simulink model "scudder"  (Simulink 2.09)
settings: Solver=ode45  StartTime=0.0  StopTime=0.4  RelTol=1e-5  AbsTol=1e-8
libraries: simulink x1
settings Model: ConsistencyChecking=off

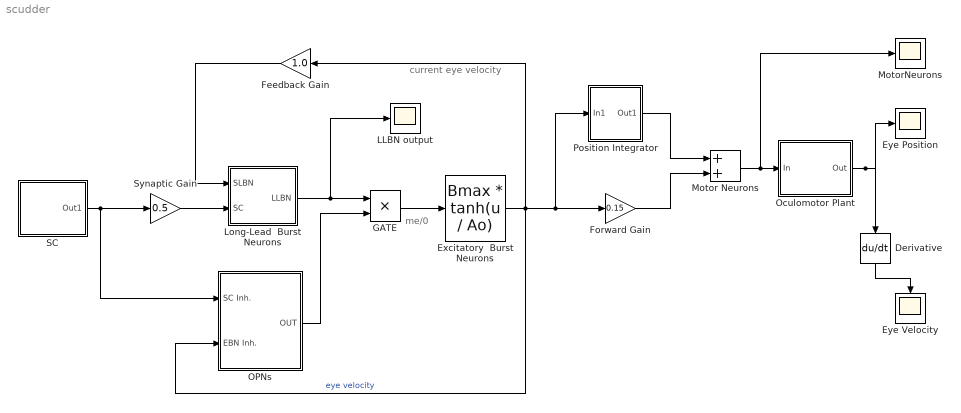
== system scudder ==
  note: current eye velocity
  note: me/0
  Derivative : Derivative  Orientation=down
  Excitatory  Burst Neurons : Fcn  Expr=Bmax * tanh(u / Ao)  mask(Burstcell Nonlinearity){Bmax=700, Ao=7}
      mask prompts: Bmax "Asymptote (Bmax): deg/s"; Ao "Angular Constant (Ao): deg"
      mask help:
      | Function:
      |        B = Bmax * tanh (me / Ao)
      |
      |     Parameters:  Bmax (deg/s)
      |                           Ao (deg)
      mask Help:
      | Bmax is the maximal firing frequency of the burst cells (expressed in deg/sec)
      |           It corresponds to the asymptote of the main sequence.
      | 
      | Ao     is the `angular constant' (in deg), which is a measure of the steepness of              the main  sequence curve for saccades.
      mask Display:
      | plot([0 1],[.5 .5]) plot([.5 .5],[0 1])
      | plot([0 .1 .2 .3 .4 .5 .6 .7 .8 .9 1],[ 0 0 .07 .17 .32 .5 .68 .83 .93 1 1])
      | text(.4,.8,'B') text(.8,.3,'me')
  Eye Position : Scope
      settings: TickLabels=on  TimeRange=auto  YMin=-10  YMax=50  SaveToWorkspace=off  SaveName=ScopeData
  Eye Velocity : Scope
      settings: Orientation=down  TickLabels=on  TimeRange=auto  YMin=-50  YMax=700  SaveToWorkspace=off  SaveName=ScopeData
  "Feedback Gain " : Gain  Orientation=left  Gain=1.0
  Forward Gain : Gain  Gain=0.15
  GATE : Product  Inputs=2
  LLBN output : Scope
      settings: TickLabels=on  TimeRange=auto  YMin=-5  YMax=20  SaveToWorkspace=off  SaveName=ScopeData
  Long-Lead  Burst Neurons : Subsystem
      mask Type: Long-Lead Burst Neurons
      mask Description: Comparator that integrates the difference between a desired eye velocity signal  from the Superior Colliculus, and the current eye velocity from the Short-Lead Burst Neurons.
      mask Display:
      | text(0.5,0.5,'LLBN')
      | text(0.05,0.8,'- slbn')
      | text(0.05,0.2,'+ SC')
  Motor Neurons : Sum  Inputs=++
  MotorNeurons : Scope
      settings: TickLabels=on  TimeRange=auto  YMin=-10  YMax=150  SaveToWorkspace=off  SaveName=ScopeData
  "OPNs " : Subsystem  mask(OPNs){DEL=15, G=0.2, bias=80}
      mask prompts: DEL "Trigger Delay (ms)"; G "SC Gain"; bias "BIAS  (Hz)"
      mask help:
      | Pause system that triggers eye by an attenuated SC input burst, and inhibits the burst generator during fixations with intensity Bias.
      | During the saccade, the burst generator inhibits the pause cells.
      mask Help:
      | User controls:
      |         Bias level (in Hz)   (defines the Pause neuron activity level during fixation)
      |         SC burst, of which the Gain can be set.
      |          Trigger delay (in ms), which determines saccade onset (and kinematics!)
      | Inputs:
      |         SC burst, attenuated by OPN inhibition gain, and delayed.
      |         Horizontal eye velocity (5ms latch delay)
      | Outputs:
      |          either 0 or 1
      mask Display:
      | plot([.1 .3],[.4 .4])
      | plot([.3 .5],[.4 .6])
      | plot([.5 .65],[.4 .4])
      | text(.65,.65,'0')
      | text(.57,.40,'me')
      | 
      | plot([.1 .7],[.3 .3])  plot([.1 .1],[.3 .7])
      | plot([.1 .7],[.7 .7])  plot([.7 .7],[.3 .7])
  Oculomotor Plant : Subsystem  mask(Oculomotor Plant){T1=0.15, T2=0.020}
      mask prompts: T1 "High Time Constant (T1)"; T2 "Low Time Constant (T2)"
      mask help:
      | Second order model of the oculomotor plant
      | as proposed by Robinson and colleagues.
      |
      |  Model equation in Laplace notation:
      |
      |                         1
      |  H(s) = ---------------
      |             (1 + s.T1) . (1 + s.T2)
      mask Help:
      | T1 is the `high' time constant (muscle twitch relaxation time)
      |       default value: 0.15 sec
      |  T2 is the `low' time constant (muscle twitch contraction time)
      |       default value: 0.012 sec
      mask Display:
      | plot([0 0.1 0.15 0.2 0.25 0.3 0.5 0.7 0.9 1], [0 0.1 0.4 0.65 0.66 0.55 0.35 0.15 0.05 0])
      | text(0.04,0.5,'T2') text(0.55,0.5, 'T1')
  Position Integrator : Subsystem  mask(Eye Position Integrator){G=1.0}
      mask prompts: G "Integrator Gain"
      mask Display: text(.35,.5,'INT')
  "SC " : Subsystem  mask{FR=800, D=50}
      mask prompts: FR "Firing Rate (FR, in Hz)"; D "Burst Duration (D,  in msec)"
      mask help: The Superior Colliculus issues a burst of spikes of height FR (Hz) and duration D (in sec).
      mask Display:
      | text(.2,.85,'SC BURST')
      | plot([.2 .35,.36,.65,.66,.8],[.05,.05,.5,.5,.05,.05])
      | text(.15,.5,'FR')
      | text(.5,.05,'D')
  Synaptic Gain : Gain  Gain=0.5
  wires:
  "SC "/1(Out1) -> "OPNs "/1(SC Inh.), Synaptic Gain/1
  Derivative/1 -> Eye Velocity/1
  Oculomotor Plant/1(Out) -> Derivative/1, Eye Position/1
  Long-Lead  Burst Neurons/1(LLBN) -> LLBN output/1, GATE/1
  GATE/1 -> Excitatory  Burst Neurons/1
  "Feedback Gain "/1 -> Long-Lead  Burst Neurons/1(SLBN)
  "OPNs "/1(OUT) -> GATE/2
  Excitatory  Burst Neurons/1 -> "Feedback Gain "/1, "OPNs "/2(EBN Inh.), Position Integrator/1(In1), Forward Gain/1  "eye velocity"
  Synaptic Gain/1 -> Long-Lead  Burst Neurons/2(SC)
  Position Integrator/1(Out1) -> Motor Neurons/1
  Forward Gain/1 -> Motor Neurons/2
  Motor Neurons/1 -> MotorNeurons/1, Oculomotor Plant/1("In ")

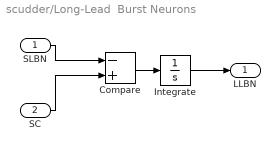
== system scudder/Long-Lead  Burst Neurons ==
  SLBN : Inport  Port=1  PortWidth=-1  SampleTime=-1
  SC : Inport  Port=2  PortWidth=-1  SampleTime=-1
  "Compare " : Sum  Inputs=-+
  Integrate : Integrator  ExternalReset=none  InitialConditionSource=internal  InitialCondition=0  LimitOutput=off  UpperSaturationLimit=inf  LowerSaturationLimit=-inf  ShowSaturationPort=off  ShowStatePort=off  AbsoluteTolerance=auto
  LLBN : Outport  Port=1  InitialOutput=0
  wires:
  SC/1 -> "Compare "/2
  Integrate/1 -> LLBN/1
  SLBN/1 -> "Compare "/1
  "Compare "/1 -> Integrate/1

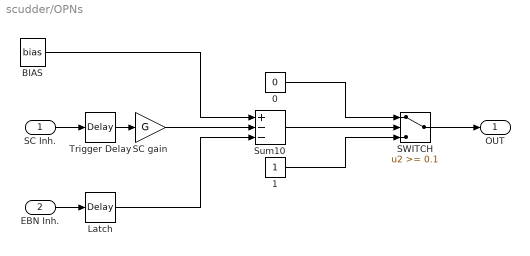
== system scudder/OPNs  ==
  SC Inh. : Inport  Port=1  PortWidth=-1  SampleTime=-1
  EBN Inh. : Inport  Port=2  PortWidth=-1  SampleTime=-1
  0 : Constant  Value=0
  1 : Constant  Value=1
  BIAS : Constant  Value=bias
  Latch : TransportDelay  DelayTime=0.005  InitialInput=0  BufferSize=1024
  SC gain : Gain  Gain=G
  SWITCH : Switch  Threshold=0.1
  Sum10 : Sum  Inputs=+--
  Trigger Delay : TransportDelay  DelayTime=0.001*DEL  InitialInput=0  BufferSize=1024
  OUT : Outport  Port=1  InitialOutput=0
  wires:
  EBN Inh./1 -> Latch/1
  Latch/1 -> Sum10/3
  Trigger Delay/1 -> SC gain/1
  SC Inh./1 -> Trigger Delay/1
  SC gain/1 -> Sum10/2
  Sum10/1 -> SWITCH/2
  1/1 -> SWITCH/3
  0/1 -> SWITCH/1
  SWITCH/1 -> OUT/1
  BIAS/1 -> Sum10/1

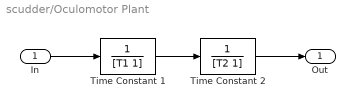
== system scudder/Oculomotor Plant ==
  "In " : Inport  Port=1  PortWidth=-1  SampleTime=-1
  Time Constant 1 : TransferFcn  Numerator=[1]  Denominator=[T1 1]
  Time Constant 2 : TransferFcn  Numerator=[1]  Denominator=[T2 1]
  Out : Outport  Port=1  InitialOutput=0
  wires:
  Time Constant 2/1 -> Out/1
  "In "/1 -> Time Constant 1/1
  Time Constant 1/1 -> Time Constant 2/1

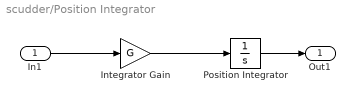
== system scudder/Position Integrator ==
  In1 : Inport  Port=1  PortWidth=-1  SampleTime=-1
  Integrator Gain : Gain  Gain=G
  Position Integrator : Integrator  ExternalReset=none  InitialConditionSource=internal  InitialCondition=0  LimitOutput=off  UpperSaturationLimit=inf  LowerSaturationLimit=-inf  ShowSaturationPort=off  ShowStatePort=off  AbsoluteTolerance=auto
  Out1 : Outport  Port=1  InitialOutput=0
  wires:
  Integrator Gain/1 -> Position Integrator/1
  Position Integrator/1 -> Out1/1
  In1/1 -> Integrator Gain/1

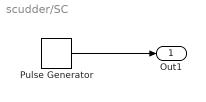
== system scudder/SC  ==
  Pulse Generator : simulink/Sources/Pulse Generator  period=1  duty=D * 0.1  amplitude=FR  start=0.05
  Out1 : Outport  Port=1  InitialOutput=0
  wires:
  Pulse Generator/1 -> Out1/1
